simulink model "Decimator"  (R2023b)
settings: Solver=VariableStepAuto  StartTime=0.0  StopTime=18000/(fclk*8)  RelTol=1e-3
PreLoadFcn:
  | startup
values from neighbouring files (symbols this model uses):
  fclk = 64e6    (= 64000000)    [startup.m]
undefined symbols (not defined in the file or in its folder): designMultirateFIR
libraries: hdlBasic x155, dspmlti4 x32, hdlsllib x2, hdlDSPIP x1, dspsrcs4 x1, vmcUtilities x1
settings Model: Creator=andre  LastModifiedBy=andre

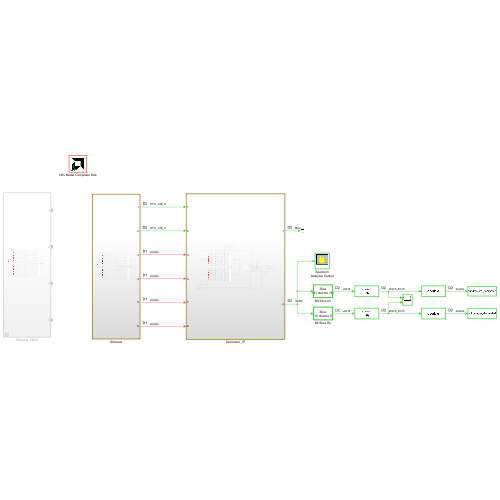
[thumbnail: Simulink's stored preview of the top-level diagram]
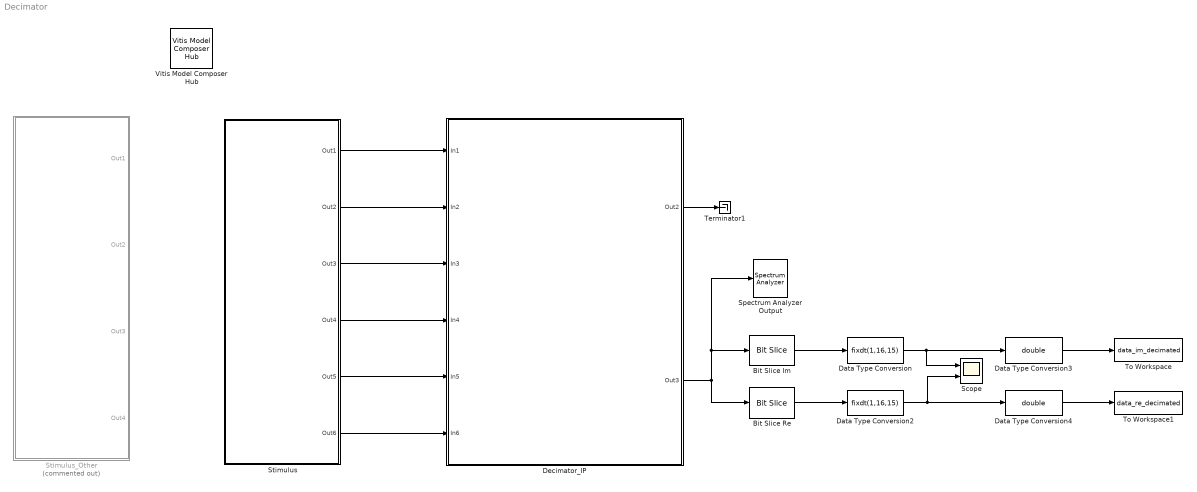
== system Decimator ==
  Bit Slice Im : hdlsllib/Logic and Bit Operations/Bit Slice  lidx=31  ridx=16
  Bit Slice Re : hdlsllib/Logic and Bit Operations/Bit Slice  lidx=15  ridx=0
  Data Type Conversion : DataTypeConversion  OutDataTypeStr=fixdt(1,16,15)  ConvertRealWorld=Stored Integer (SI)  SaturateOnIntegerOverflow=off  RndMeth=Floor
  Data Type Conversion2 : DataTypeConversion  OutDataTypeStr=fixdt(1,16,15)  ConvertRealWorld=Stored Integer (SI)  SaturateOnIntegerOverflow=off  RndMeth=Floor
  Data Type Conversion3 : DataTypeConversion  OutDataTypeStr=double  RndMeth=Floor
  Data Type Conversion4 : DataTypeConversion  OutDataTypeStr=double  RndMeth=Floor
  Decimator_IP : Subsystem
  Scope : Scope  NumInputPorts=2
  Spectrum Analyzer Output : SpectrumAnalyzer  WindowPosition=[2932.000000,-90.000000,799.000000,500.000000,]  ScopeFrameLocation=window  Span=64000000  StartFrequency=-32000000  StopFrequency=32000000  YLimits=[41.6132,126.1267]  SelectedToolstripTab=spectrumAnalyzerToolstrip.measurementsTab
  Stimulus : Subsystem
  Stimulus_Other : Subsystem  Commented=on
  Terminator1 : Terminator
  To Workspace : ToWorkspace  VariableName=data_im_decimated  SaveFormat=Timeseries  SampleTime=-1
  To Workspace1 : ToWorkspace  VariableName=data_re_decimated  SaveFormat=Timeseries  SampleTime=-1
  Vitis Model Composer Hub : vmcUtilities/Vitis Model Composer Hub  Tag=genX  CodeGeneration=off  SubsystemName=Decimator_IP  DUTSubsystemName=Decimator_IP  CompilationType=HDLCompilation  ExportTypeV2=IP Catalog  TargetDirectory=./netlist\ip\Decimator_IP\src  exportDesign=on  analyzeDesign=off  validateDesignOnHw=off  ExportType=HDL  IpVendor=xilinx.com  IpLibrary=hls  IpVersion=1.0  IpHWLanguage=Verilog  AieCompilerOptions={}  AieSimulatorOptions={}  CreateTestbench=off  TestbenchStackSize=10  RunRtlSim=off  RunCSim=off  RunAieSim=off  AieSimTimeout=50000  RunAieSimProfiling=off  LaunchVitisAnalyzer=off  PlotOutput=off  RunX86Sim=off  X86SimTimeout=10  GenHwImage=off  GenLibadfXo=on  GenHwValidationCode=off  PlatformType=Not Specified  HwSystemType=Baremetal  HwValidationTarget=hw  ProjDevice=xczu28dr-ffvg1517-2-e  ProjDevicePart=xczu28dr-ffvg1517-2-e  SamplePeriod=-1  ClockFrequency=200  DataPathParallelism=1  xilinxfamily=zynquplusRFSOC  part=xczu28dr  speed=-2-e  package=ffvg1517  directory=./netlist\ip\Decimator_IP\src  testbench=off  incr_netlist=off  synthesis_tool=Vivado  clock_wrapper=Clock Enables  dbl_ovrd=According to Block Masks  dcm_input_clock_period=10  sysclk_period=(1/fclk)*(1e6)  simulink_period=1/(fclk*8)  eval_field=0  IPInfoJsonString="{\"HDLSubsystem\":{\"SubsystemName\":\"Decimator_IP\",\"IPName\":\"Decimator\",\"IPLibrary\":\"VMC\",\"IPVendor\":\"CoRSoC\",\"IPVersion\":\"1.0\",\"TargetDirectory\":\"./netlist\",\"SubsystemDir\":\"./netlist\\\\ip\\\\Decimator_IP\"},\"SubsystemTag\":\"HDLNode\"}"  LogFileName=''  NThreads=4
  wires:
  Decimator_IP/1(Out2) -> Terminator1/1
  Data Type Conversion3/1 -> To Workspace/1
  Data Type Conversion4/1 -> To Workspace1/1
  Stimulus/1(Out1) -> Decimator_IP/1(In1)
  Stimulus/2(Out2) -> Decimator_IP/2(In2)
  Decimator_IP/2(Out3) -> Bit Slice Im/1, Spectrum Analyzer Output/1, Bit Slice Re/1
  Bit Slice Im/1 -> Data Type Conversion/1
  Bit Slice Re/1 -> Data Type Conversion2/1
  Stimulus/3(Out3) -> Decimator_IP/3(In3)
  Stimulus/4(Out4) -> Decimator_IP/4(In4)
  Data Type Conversion/1 -> Data Type Conversion3/1, Scope/1
  Data Type Conversion2/1 -> Scope/2, Data Type Conversion4/1
  Stimulus/5(Out5) -> Decimator_IP/5(In5)
  Stimulus/6(Out6) -> Decimator_IP/6(In6)

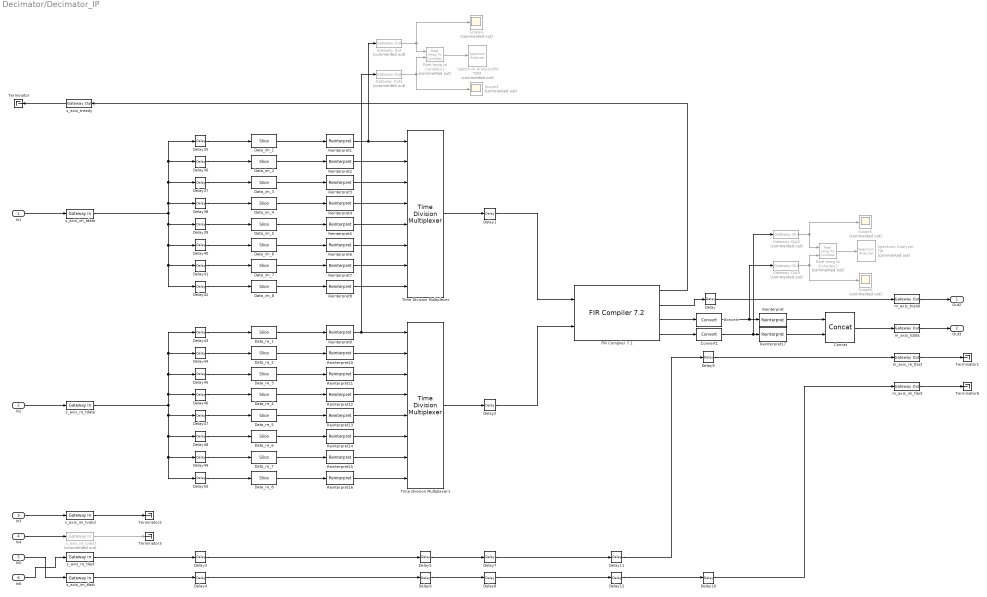
== system Decimator/Decimator_IP ==
  In1 : Inport
  In2 : Inport  Port=2
  In3 : Inport  Port=3
  In4 : Inport  Port=4
  In5 : Inport  Port=5
  In6 : Inport  Port=6
  Concat : hdlBasic/Concat  num_inputs=2  XmcBlockStatus=1  maskContainerNames=group1  block_type=concat  block_config=sysgen:Concat_config
  Convert : hdlBasic/Convert  gui_display_data_type=Fixed-point  arith_type=Signed (2's comp)  n_bits=16  bin_pt=15  float_type=Single  exp_bits=8  fraction_bits=24  quantization=Truncate  overflow=Saturate  en=off  latency=1  pipeline=off  XmcBlockStatus=1  maskContainerNames=group2  block_type=convert  block_config=sysgen:Convert_config  block_width=595  block_height=885
  Convert1 : hdlBasic/Convert  gui_display_data_type=Fixed-point  arith_type=Signed (2's comp)  n_bits=16  bin_pt=15  float_type=Single  exp_bits=8  fraction_bits=24  quantization=Truncate  overflow=Saturate  en=off  latency=1  pipeline=off  XmcBlockStatus=1  maskContainerNames=group2  block_type=convert  block_config=sysgen:Convert_config  block_width=595  block_height=885
  Data_im_1 : hdlBasic/Slice  nbits=16  boolean_output=off  mode=Upper Bit Location + Width  bit1=127  base1=LSB of Input  bit0=16*8-(16*1)  base0=LSB of Input  XmcBlockStatus=1  maskContainerNames=group1  block_type=slice  block_config=sysgen:Slice_config
  Data_im_2 : hdlBasic/Slice  nbits=16  boolean_output=off  mode=Upper Bit Location + Width  bit1=111  base1=LSB of Input  bit0=16*8-(16*1)  base0=LSB of Input  XmcBlockStatus=1  maskContainerNames=group1  block_type=slice  block_config=sysgen:Slice_config
  Data_im_3 : hdlBasic/Slice  nbits=16  boolean_output=off  mode=Upper Bit Location + Width  bit1=95  base1=LSB of Input  bit0=16*8-(16*1)  base0=LSB of Input  XmcBlockStatus=1  maskContainerNames=group1  block_type=slice  block_config=sysgen:Slice_config
  Data_im_4 : hdlBasic/Slice  nbits=16  boolean_output=off  mode=Upper Bit Location + Width  bit1=79  base1=LSB of Input  bit0=16*8-(16*1)  base0=LSB of Input  XmcBlockStatus=1  maskContainerNames=group1  block_type=slice  block_config=sysgen:Slice_config
  Data_im_5 : hdlBasic/Slice  nbits=16  boolean_output=off  mode=Upper Bit Location + Width  bit1=63  base1=LSB of Input  bit0=16*8-(16*1)  base0=LSB of Input  XmcBlockStatus=1  maskContainerNames=group1  block_type=slice  block_config=sysgen:Slice_config
  Data_im_6 : hdlBasic/Slice  nbits=16  boolean_output=off  mode=Upper Bit Location + Width  bit1=47  base1=LSB of Input  bit0=16*8-(16*1)  base0=LSB of Input  XmcBlockStatus=1  maskContainerNames=group1  block_type=slice  block_config=sysgen:Slice_config
  Data_im_7 : hdlBasic/Slice  nbits=16  boolean_output=off  mode=Upper Bit Location + Width  bit1=31  base1=LSB of Input  bit0=16*8-(16*1)  base0=LSB of Input  XmcBlockStatus=1  maskContainerNames=group1  block_type=slice  block_config=sysgen:Slice_config
  Data_im_8 : hdlBasic/Slice  nbits=16  boolean_output=off  mode=Upper Bit Location + Width  bit1=15  base1=LSB of Input  bit0=16*8-(16*1)  base0=LSB of Input  XmcBlockStatus=1  maskContainerNames=group1  block_type=slice  block_config=sysgen:Slice_config
  Data_re_1 : hdlBasic/Slice  nbits=16  boolean_output=off  mode=Upper Bit Location + Width  bit1=127  base1=LSB of Input  bit0=16*8-(16*1)  base0=LSB of Input  XmcBlockStatus=1  maskContainerNames=group1  block_type=slice  block_config=sysgen:Slice_config
  Data_re_2 : hdlBasic/Slice  nbits=16  boolean_output=off  mode=Upper Bit Location + Width  bit1=111  base1=LSB of Input  bit0=16*8-(16*1)  base0=LSB of Input  XmcBlockStatus=1  maskContainerNames=group1  block_type=slice  block_config=sysgen:Slice_config
  Data_re_3 : hdlBasic/Slice  nbits=16  boolean_output=off  mode=Upper Bit Location + Width  bit1=95  base1=LSB of Input  bit0=16*8-(16*1)  base0=LSB of Input  XmcBlockStatus=1  maskContainerNames=group1  block_type=slice  block_config=sysgen:Slice_config
  Data_re_4 : hdlBasic/Slice  nbits=16  boolean_output=off  mode=Upper Bit Location + Width  bit1=79  base1=LSB of Input  bit0=16*8-(16*1)  base0=LSB of Input  XmcBlockStatus=1  maskContainerNames=group1  block_type=slice  block_config=sysgen:Slice_config
  Data_re_5 : hdlBasic/Slice  nbits=16  boolean_output=off  mode=Upper Bit Location + Width  bit1=63  base1=LSB of Input  bit0=16*8-(16*1)  base0=LSB of Input  XmcBlockStatus=1  maskContainerNames=group1  block_type=slice  block_config=sysgen:Slice_config
  Data_re_6 : hdlBasic/Slice  nbits=16  boolean_output=off  mode=Upper Bit Location + Width  bit1=47  base1=LSB of Input  bit0=16*8-(16*1)  base0=LSB of Input  XmcBlockStatus=1  maskContainerNames=group1  block_type=slice  block_config=sysgen:Slice_config
  Data_re_7 : hdlBasic/Slice  nbits=16  boolean_output=off  mode=Upper Bit Location + Width  bit1=31  base1=LSB of Input  bit0=16*8-(16*1)  base0=LSB of Input  XmcBlockStatus=1  maskContainerNames=group1  block_type=slice  block_config=sysgen:Slice_config
  Data_re_8 : hdlBasic/Slice  nbits=16  boolean_output=off  mode=Upper Bit Location + Width  bit1=15  base1=LSB of Input  bit0=16*8-(16*1)  base0=LSB of Input  XmcBlockStatus=1  maskContainerNames=group1  block_type=slice  block_config=sysgen:Slice_config
  Delay{,1..4,7..10,35..50} (25 alike) : hdlBasic/Delay  rst=off  en=off  latency=1  reg_retiming=off  XmcBlockStatus=1  maskContainerNames=group1  block_type=delay  block_config=sysgen:Delay_config
  Delay11 : hdlBasic/Delay  rst=off  en=off  latency=6  reg_retiming=off  XmcBlockStatus=1  maskContainerNames=group1  block_type=delay  block_config=sysgen:Delay_config
  Delay12 : hdlBasic/Delay  rst=off  en=off  latency=6  reg_retiming=off  XmcBlockStatus=1  maskContainerNames=group1  block_type=delay  block_config=sysgen:Delay_config
  Delay5 : hdlBasic/Delay  rst=off  en=off  latency=7  reg_retiming=off  XmcBlockStatus=1  maskContainerNames=group1  block_type=delay  block_config=sysgen:Delay_config
  Delay6 : hdlBasic/Delay  rst=off  en=off  latency=7  reg_retiming=off  XmcBlockStatus=1  maskContainerNames=group1  block_type=delay  block_config=sysgen:Delay_config
  FIR Compiler 7.1 : hdlDSPIP/FIR Compiler 7.2   coefficientvector=coeffs  coefficient_sets=1  coefficient_reload=off  filter_type=Decimation  rate_change_type=Integer  interpolation_rate=1  decimation_rate=8  zero_pack_factor=1  channel_sequence=Basic  number_channels=1  pattern_list='P4-0,P4-1,P4-2,P4-3,P4-4'  number_paths=2  ratespecification=Maximum_Possible  sampleperiod=1  hardwareoversamplingrate=1  coefficient_sign=Signed  quantization=Quantize_Only  coefficient_width=16  bestprecision=on  coefficient_fractional_bits=17  coefficient_structure=Inferred  output_rounding_mode=Full_Precision  output_width=35  filter_architecture=Systolic_Multiply_Accumulate  optimization_goal=Speed  optimization_list='Data_Path_Fanout,Pre-Adder_Pipeline,Coefficient_Fanout,Control_Path_Fanout,Control_Column_Fanout,Control_Broadcast_Fanout,Control_LUT_Pipeline,No_BRAM_Read_First_Mode,Optimal_Column_Lengths,Other'  data_buffer_type=Automatic  coefficient_buffer_type=Automatic  input_buffer_type=Automatic  output_buffer_type=Automatic  preference_for_other_storage=Automatic  multi_column_support=Automatic  columnconfig='15'  inter_column_pipe_length=4  data_has_tlast=Not_Required  m_data_has_tready=off  s_data_has_fifo=off  s_data_has_tuser=Not_Required  m_data_has_tuser=Not_Required  s_config_sync_mode=On_Vector  s_config_method=Single  num_reload_slots=1  has_aclken=off  has_aresetn=off  reset_data_vector=on  trim_axipin_name=on  simulation_type=hybrid_sim  simulation_model=sysgen:xfirv7_2_cmodel  data_path_portlist={ 's_axis_data_tdata', 'm_axis_data_tdata' }  passband_min=0.0  passband_max=0.5  stopband_min=0.5  stopband_max=1.0  filter_selection=1  gui_behaviour='Sysgen_GUI'  data_sign=Signed  data_width=16  data_fractional_bits=0  data_tuser_width=1  wrapper_available=true  ip_wrap_arbitrary_binary_point=true  ip_name=FIR Compiler  ip_version=7.2  dsptool_ready=true  ipcore_usecache=true  ipcore_useipmodelcache=true  port_translation_map={ 'aclken' => 'en', 'aresetn' => 'rst' }  run_core_at_system_period=true  ipcore_xco_need_fpga_part=true  ipcore_fpga_part=[]  XmcBlockStatus=1  maskContainerNames=tabcontainer1  block_type=fir_compiler_v7_2  block_config=sysgen:rodinimport_config  block_width=820  block_height=600
  Gateway Out{,1..3} (4 alike) : hdlBasic/Gateway Out  Commented=on  inherit_from_input=off  hdl_port=off  rows=1  columns=1  UseAsDAC=off  DACChannel='1'  interface=None  automatic_assignment=on  address_offset=hex2dec('00')  intf_name=''  intf_description=''  timing_constraint=None  locs_specified=off  LOCs={}  io_standard={}  XmcBlockStatus=1  maskContainerNames=group4  block_type=gatewayout  block_config=sysgen:gateway_out_config  block_width_w=590  block_height_w=620  block_width=620  block_height=750
  Real-Imag to Complex1 : RealImagToComplex  Commented=on
  Real-Imag to Complex2 : RealImagToComplex  Commented=on
  Reinterpret : hdlBasic/Reinterpret  force_arith_type=on  arith_type=Unsigned  force_bin_pt=on  bin_pt=0  XmcBlockStatus=1  maskContainerNames=group1  block_type=reinterpret  block_config=sysgen:Reinterpret_config
  Reinterpret{1..16} (16 alike) : hdlBasic/Reinterpret  force_arith_type=on  arith_type="Signed  (2's comp)"  force_bin_pt=on  bin_pt=15  XmcBlockStatus=1  maskContainerNames=group1  block_type=reinterpret  block_config=sysgen:Reinterpret_config
  Reinterpret17 : hdlBasic/Reinterpret  force_arith_type=on  arith_type=Unsigned  force_bin_pt=on  bin_pt=0  XmcBlockStatus=1  maskContainerNames=group1  block_type=reinterpret  block_config=sysgen:Reinterpret_config
  Scope{3..6} (4 alike) : Scope  Commented=on
  Spectrum Analyzer FIR : SpectrumAnalyzer  Commented=on  WindowPosition=[481.000000,-215.000000,800.000000,500.000000,]  ScopeFrameLocation=window  Span=64000000  StartFrequency=-32000000  StopFrequency=32000000  YLimits=[-174.72319427,-62.57953967]  SelectedToolstripTab=spectrumAnalyzerToolstrip.measurementsTab
  Spectrum AnalyzerB4 TDM : SpectrumAnalyzer  Commented=on  WindowPosition=[274.000000,72.000000,800.000000,500.000000,]  ScopeFrameLocation=window  Span=512000000  StartFrequency=-256000000  StopFrequency=256000000  YLimits=[-191.4141624,-56.39167641]  SelectedToolstripTab=spectrumAnalyzerToolstrip.measurementsTab
  Terminator{,1..3,6} (5 alike) : Terminator
  Time Division Multiplexer : hdlBasic/Time Division Multiplexer  inputs=8  vin=off  Optimization=Speed  explicit_period=off  period=1  XmcBlockStatus=1  maskContainerNames=group3  block_type=tdm  block_config=sysgen:TDM_config
  Time Division Multiplexer1 : hdlBasic/Time Division Multiplexer  inputs=8  vin=off  Optimization=Speed  explicit_period=off  period=1  XmcBlockStatus=1  maskContainerNames=group3  block_type=tdm  block_config=sysgen:TDM_config
  m_axis_im_tlast : hdlBasic/Gateway Out  inherit_from_input=off  hdl_port=on  rows=1  columns=1  UseAsDAC=off  DACChannel='1'  interface=None  automatic_assignment=on  address_offset=hex2dec('00')  intf_name=''  intf_description=''  timing_constraint=None  locs_specified=off  LOCs={}  io_standard={}  XmcBlockStatus=1  maskContainerNames=group4  block_type=gatewayout  block_config=sysgen:gateway_out_config  block_width_w=590  block_height_w=620  block_width=620  block_height=750
  m_axis_re_tlast : hdlBasic/Gateway Out  inherit_from_input=off  hdl_port=on  rows=1  columns=1  UseAsDAC=off  DACChannel='1'  interface=None  automatic_assignment=on  address_offset=hex2dec('00')  intf_name=''  intf_description=''  timing_constraint=None  locs_specified=off  LOCs={}  io_standard={}  XmcBlockStatus=1  maskContainerNames=group4  block_type=gatewayout  block_config=sysgen:gateway_out_config  block_width_w=590  block_height_w=620  block_width=620  block_height=750
  m_axis_tdata : hdlBasic/Gateway Out  inherit_from_input=on  hdl_port=on  rows=1  columns=1  UseAsDAC=off  DACChannel='1'  interface=None  automatic_assignment=on  address_offset=hex2dec('00')  intf_name=''  intf_description=''  timing_constraint=None  locs_specified=off  LOCs={}  io_standard={}  XmcBlockStatus=1  maskContainerNames=group4  block_type=gatewayout  block_config=sysgen:gateway_out_config  block_width_w=590  block_height_w=620  block_width=620  block_height=750
  m_axis_tvalid : hdlBasic/Gateway Out  inherit_from_input=off  hdl_port=on  rows=1  columns=1  UseAsDAC=off  DACChannel='1'  interface=None  automatic_assignment=on  address_offset=hex2dec('00')  intf_name=''  intf_description=''  timing_constraint=None  locs_specified=off  LOCs={}  io_standard={}  XmcBlockStatus=1  maskContainerNames=group4  block_type=gatewayout  block_config=sysgen:gateway_out_config  block_width_w=590  block_height_w=620  block_width=620  block_height=750
  s_axis_im_tdata : hdlBasic/Gateway In  gui_display_data_type=Fixed-point  arith_type=Unsigned  n_bits=16*8  bin_pt=0  preci_type=Single  exp_width=8  frac_width=24  rows=1  columns=1  quantization=Truncate  overflow=Saturate  period=1/fclk  UseAsADC=off  ADCChannel='1'  interface=None  automatic_assignment=on  address_offset=hex2dec('00')  intf_name=''  intf_description=''  default_value=0  timing_constraint=None  locs_specified=off  LOCs={}  io_standard={}  inherit_from_input=off  hdl_port=on  XmcBlockStatus=1  maskContainerNames=group4  block_type=gatewayin  block_config=sysgen:gateway_in_config  block_width_w=590  block_height_w=620  block_width=640  block_height=850
  s_axis_im_tlast : hdlBasic/Gateway In  gui_display_data_type=Boolean  arith_type=Boolean  n_bits=32  bin_pt=0  preci_type=Single  exp_width=8  frac_width=24  rows=1  columns=1  quantization="Round  (unbiased: +/- Inf)"  overflow=Saturate  period=1/fclk  UseAsADC=off  ADCChannel='1'  interface=None  automatic_assignment=on  address_offset=hex2dec('00')  intf_name=''  intf_description=''  default_value=0  timing_constraint=None  locs_specified=off  LOCs={}  io_standard={}  inherit_from_input=off  hdl_port=on  XmcBlockStatus=1  maskContainerNames=group4  block_type=gatewayin  block_config=sysgen:gateway_in_config  block_width_w=590  block_height_w=620  block_width=640  block_height=850
  s_axis_im_tvalid : hdlBasic/Gateway In  gui_display_data_type=Boolean  arith_type=Boolean  n_bits=32  bin_pt=0  preci_type=Single  exp_width=8  frac_width=24  rows=1  columns=1  quantization="Round  (unbiased: +/- Inf)"  overflow=Saturate  period=1/fclk  UseAsADC=off  ADCChannel='1'  interface=None  automatic_assignment=on  address_offset=hex2dec('00')  intf_name=''  intf_description=''  default_value=0  timing_constraint=None  locs_specified=off  LOCs={}  io_standard={}  inherit_from_input=off  hdl_port=on  XmcBlockStatus=1  maskContainerNames=group4  block_type=gatewayin  block_config=sysgen:gateway_in_config  block_width_w=590  block_height_w=620  block_width=640  block_height=850
  s_axis_re_tdata : hdlBasic/Gateway In  gui_display_data_type=Fixed-point  arith_type=Unsigned  n_bits=16*8  bin_pt=0  preci_type=Single  exp_width=8  frac_width=24  rows=1  columns=1  quantization=Truncate  overflow=Saturate  period=1/fclk  UseAsADC=off  ADCChannel='1'  interface=None  automatic_assignment=on  address_offset=hex2dec('00')  intf_name=''  intf_description=''  default_value=0  timing_constraint=None  locs_specified=off  LOCs={}  io_standard={}  inherit_from_input=off  hdl_port=on  XmcBlockStatus=1  maskContainerNames=group4  block_type=gatewayin  block_config=sysgen:gateway_in_config  block_width_w=590  block_height_w=620  block_width=640  block_height=850
  s_axis_re_tlast : hdlBasic/Gateway In  gui_display_data_type=Boolean  arith_type=Boolean  n_bits=32  bin_pt=0  preci_type=Single  exp_width=8  frac_width=24  rows=1  columns=1  quantization="Round  (unbiased: +/- Inf)"  overflow=Saturate  period=1/fclk  UseAsADC=off  ADCChannel='1'  interface=None  automatic_assignment=on  address_offset=hex2dec('00')  intf_name=''  intf_description=''  default_value=0  timing_constraint=None  locs_specified=off  LOCs={}  io_standard={}  inherit_from_input=off  hdl_port=on  XmcBlockStatus=1  maskContainerNames=group4  block_type=gatewayin  block_config=sysgen:gateway_in_config  block_width_w=590  block_height_w=620  block_width=640  block_height=850
  s_axis_re_tvalid : hdlBasic/Gateway In  Commented=on  gui_display_data_type=Boolean  arith_type=Boolean  n_bits=32  bin_pt=0  preci_type=Single  exp_width=8  frac_width=24  rows=1  columns=1  quantization="Round  (unbiased: +/- Inf)"  overflow=Saturate  period=1/fclk  UseAsADC=off  ADCChannel='1'  interface=None  automatic_assignment=on  address_offset=hex2dec('00')  intf_name=''  intf_description=''  default_value=0  timing_constraint=None  locs_specified=off  LOCs={}  io_standard={}  inherit_from_input=off  hdl_port=on  XmcBlockStatus=1  maskContainerNames=group4  block_type=gatewayin  block_config=sysgen:gateway_in_config  block_width_w=590  block_height_w=620  block_width=640  block_height=850
  s_axis_tready : hdlBasic/Gateway Out  inherit_from_input=off  hdl_port=on  rows=1  columns=1  UseAsDAC=off  DACChannel='1'  interface=None  automatic_assignment=on  address_offset=hex2dec('00')  intf_name=''  intf_description=''  timing_constraint=None  locs_specified=off  LOCs={}  io_standard={}  XmcBlockStatus=1  maskContainerNames=group4  block_type=gatewayout  block_config=sysgen:gateway_out_config  block_width_w=590  block_height_w=620  block_width=620  block_height=750
  Out2 : Outport
  Out3 : Outport  Port=2
  wires:
  In2/1 -> s_axis_re_tdata/1
  In1/1 -> s_axis_im_tdata/1
  FIR Compiler 7.1/2 -> Delay/1
  FIR Compiler 7.1/3 -> Convert/1
  Reinterpret17/1 -> Concat/2
  Convert/1 -> Gateway Out3/1, Reinterpret/1
  FIR Compiler 7.1/1 -> s_axis_tready/1
  Delay/1 -> m_axis_tvalid/1
  Convert1/1 -> Gateway Out2/1, Reinterpret17/1
  Concat/1 -> m_axis_tdata/1
  FIR Compiler 7.1/4 -> Convert1/1
  Reinterpret/1 -> Concat/1
  s_axis_im_tdata/1 -> Delay42/1, Delay41/1, Delay40/1, Delay39/1, Delay38/1, Delay37/1, Delay36/1, Delay35/1
  s_axis_re_tdata/1 -> Delay50/1, Delay49/1, Delay48/1, Delay47/1, Delay46/1, Delay45/1, Delay43/1, Delay44/1
  s_axis_re_tvalid/1 -> Terminator3/1
  s_axis_im_tvalid/1 -> Terminator2/1
  In3/1 -> s_axis_im_tvalid/1
  In4/1 -> s_axis_re_tvalid/1
  s_axis_tready/1 -> Terminator/1
  Time Division Multiplexer/1 -> Delay1/1
  Delay1/1 -> FIR Compiler 7.1/1
  Time Division Multiplexer1/1 -> Delay2/1
  Delay2/1 -> FIR Compiler 7.1/2
  Data_im_1/1 -> Reinterpret1/1
  Data_im_2/1 -> Reinterpret2/1
  Data_im_3/1 -> Reinterpret3/1
  Data_im_4/1 -> Reinterpret4/1
  Data_im_6/1 -> Reinterpret6/1
  Data_im_7/1 -> Reinterpret7/1
  Data_im_8/1 -> Reinterpret8/1
  Data_im_5/1 -> Reinterpret5/1
  Data_re_1/1 -> Reinterpret9/1
  Data_re_3/1 -> Reinterpret11/1
  Data_re_8/1 -> Reinterpret16/1
  Data_re_6/1 -> Reinterpret14/1
  Data_re_7/1 -> Reinterpret15/1
  Data_re_4/1 -> Reinterpret12/1
  Data_re_2/1 -> Reinterpret10/1
  Data_re_5/1 -> Reinterpret13/1
  Reinterpret7/1 -> Time Division Multiplexer/7
  Reinterpret2/1 -> Time Division Multiplexer/2
  Reinterpret8/1 -> Time Division Multiplexer/8
  Reinterpret6/1 -> Time Division Multiplexer/6
  Reinterpret3/1 -> Time Division Multiplexer/3
  Reinterpret4/1 -> Time Division Multiplexer/4
  Reinterpret5/1 -> Time Division Multiplexer/5
  Reinterpret15/1 -> Time Division Multiplexer1/7
  Reinterpret14/1 -> Time Division Multiplexer1/6
  Reinterpret12/1 -> Time Division Multiplexer1/4
  Reinterpret11/1 -> Time Division Multiplexer1/3
  Reinterpret10/1 -> Time Division Multiplexer1/2
  Reinterpret13/1 -> Time Division Multiplexer1/5
  Reinterpret16/1 -> Time Division Multiplexer1/8
  Delay35/1 -> Data_im_1/1
  Delay36/1 -> Data_im_2/1
  Delay37/1 -> Data_im_3/1
  Delay38/1 -> Data_im_4/1
  Delay39/1 -> Data_im_5/1
  Delay40/1 -> Data_im_6/1
  Delay41/1 -> Data_im_7/1
  Delay42/1 -> Data_im_8/1
  Delay43/1 -> Data_re_1/1
  Delay44/1 -> Data_re_2/1
  Delay45/1 -> Data_re_3/1
  Delay46/1 -> Data_re_4/1
  Delay47/1 -> Data_re_5/1
  Delay48/1 -> Data_re_6/1
  Delay49/1 -> Data_re_7/1
  Delay50/1 -> Data_re_8/1
  m_axis_tvalid/1 -> Out2/1
  m_axis_tdata/1 -> Out3/1
  Real-Imag to Complex1/1 -> Spectrum AnalyzerB4 TDM/1
  Reinterpret9/1 -> Time Division Multiplexer1/1, Gateway Out1/1
  Gateway Out/1 -> Scope4/1, Real-Imag to Complex1/1
  Gateway Out1/1 -> Real-Imag to Complex1/2, Scope3/1
  Reinterpret1/1 -> Time Division Multiplexer/1, Gateway Out/1
  Gateway Out2/1 -> Scope5/1, Real-Imag to Complex2/1
  Gateway Out3/1 -> Scope6/1, Real-Imag to Complex2/2
  Real-Imag to Complex2/1 -> Spectrum Analyzer FIR/1
  m_axis_re_tlast/1 -> Terminator1/1
  s_axis_re_tlast/1 -> Delay3/1
  s_axis_im_tlast/1 -> Delay4/1
  m_axis_im_tlast/1 -> Terminator6/1
  In5/1 -> s_axis_im_tlast/1
  In6/1 -> s_axis_re_tlast/1
  Delay3/1 -> Delay5/1
  Delay4/1 -> Delay6/1
  Delay5/1 -> Delay7/1
  Delay6/1 -> Delay8/1
  Delay7/1 -> Delay11/1
  Delay8/1 -> Delay12/1
  Delay9/1 -> m_axis_re_tlast/1
  Delay10/1 -> m_axis_im_tlast/1
  Delay11/1 -> Delay9/1
  Delay12/1 -> Delay10/1

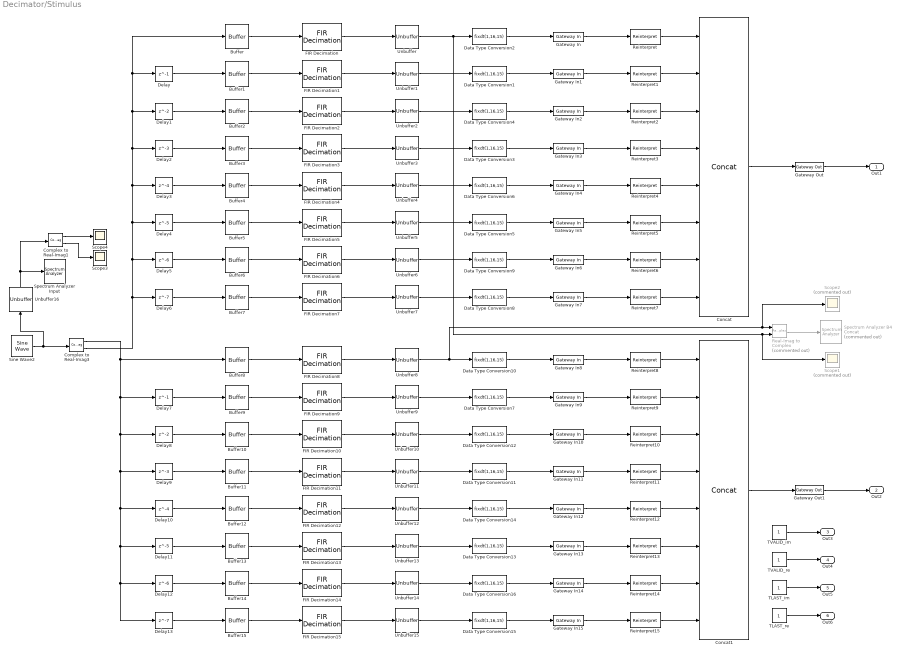
== system Decimator/Stimulus ==
  Buffer{,1..15} (16 alike) : Buffer  OutputFrames=off
  Complex to Real-Imag1 : ComplexToRealImag
  Complex to Real-Imag3 : ComplexToRealImag
  Concat : hdlBasic/Concat  num_inputs=8  XmcBlockStatus=1  maskContainerNames=group1  block_type=concat  block_config=sysgen:Concat_config
  Concat1 : hdlBasic/Concat  num_inputs=8  XmcBlockStatus=1  maskContainerNames=group1  block_type=concat  block_config=sysgen:Concat_config
  Data Type Conversion{1..16} (16 alike) : DataTypeConversion  OutDataTypeStr=fixdt(1,16,15)  RndMeth=Floor
  Delay : Delay  DelayLength=1  InitialCondition=0
  Delay1 : Delay  InitialCondition=0
  Delay10 : Delay  DelayLength=4  InitialCondition=0
  Delay11 : Delay  DelayLength=5  InitialCondition=0
  Delay12 : Delay  DelayLength=6  InitialCondition=0
  Delay13 : Delay  DelayLength=7  InitialCondition=0
  Delay2 : Delay  DelayLength=3  InitialCondition=0
  Delay3 : Delay  DelayLength=4  InitialCondition=0
  Delay4 : Delay  DelayLength=5  InitialCondition=0
  Delay5 : Delay  DelayLength=6  InitialCondition=0
  Delay6 : Delay  DelayLength=7  InitialCondition=0
  Delay7 : Delay  DelayLength=1  InitialCondition=0
  Delay8 : Delay  InitialCondition=0
  Delay9 : Delay  DelayLength=3  InitialCondition=0
  FIR Decimation{,1..15} (16 alike) : dspmlti4/FIR Decimation  FilterSource=Auto  h=designMultirateFIR(1,2)  D=8  filtStruct=Direct form  FilterObject=FDECIM  InputProcessing=Columns as channels (frame based)  framing=Enforce single-rate processing  AllowArbitraryInputLength=off  inputOffset=0  outputBufInitCond=0  roundingMode=Floor  overflowMode=on  firstCoeffDataTypeStr=Inherit: Same word length as input  firstCoeffMin=[]  firstCoeffMax=[]  firstCoeffLastDataTypeStr=Inherit: Same word length as input  outputDataTypeStr=Inherit: Same as accumulator  outputMin=[]  outputMax=[]  outputLastDataTypeStr=Inherit: Same as accumulator
  Gateway In{,1..15} (16 alike) : hdlBasic/Gateway In  gui_display_data_type=Fixed-point  arith_type=Signed (2's comp)  n_bits=16  bin_pt=15  preci_type=Single  exp_width=8  frac_width=24  rows=1  columns=1  quantization=Truncate  overflow=Saturate  period=1/(fclk)  UseAsADC=off  ADCChannel='1'  interface=None  automatic_assignment=on  address_offset=hex2dec('00')  intf_name=''  intf_description=''  default_value=0  timing_constraint=None  locs_specified=off  LOCs={}  io_standard={}  inherit_from_input=off  hdl_port=on  XmcBlockStatus=1  maskContainerNames=group4  block_type=gatewayin  block_config=sysgen:gateway_in_config  block_width_w=590  block_height_w=620  block_width=640  block_height=850
  Gateway Out : hdlBasic/Gateway Out  inherit_from_input=on  hdl_port=off  rows=1  columns=1  UseAsDAC=off  DACChannel='1'  interface=None  automatic_assignment=on  address_offset=hex2dec('00')  intf_name=''  intf_description=''  timing_constraint=None  locs_specified=off  LOCs={}  io_standard={}  XmcBlockStatus=1  maskContainerNames=group4  block_type=gatewayout  block_config=sysgen:gateway_out_config  block_width_w=590  block_height_w=620  block_width=620  block_height=750
  Gateway Out1 : hdlBasic/Gateway Out  inherit_from_input=on  hdl_port=off  rows=1  columns=1  UseAsDAC=off  DACChannel='1'  interface=None  automatic_assignment=on  address_offset=hex2dec('00')  intf_name=''  intf_description=''  timing_constraint=None  locs_specified=off  LOCs={}  io_standard={}  XmcBlockStatus=1  maskContainerNames=group4  block_type=gatewayout  block_config=sysgen:gateway_out_config  block_width_w=590  block_height_w=620  block_width=620  block_height=750
  Real-Imag to Complex : RealImagToComplex  Commented=on
  Reinterpret{,1..15} (16 alike) : hdlBasic/Reinterpret  force_arith_type=on  arith_type=Unsigned  force_bin_pt=on  bin_pt=0  XmcBlockStatus=1  maskContainerNames=group1  block_type=reinterpret  block_config=sysgen:Reinterpret_config
  Scope1 : Scope  Commented=on
  Scope2 : Scope  Commented=on
  Scope3 : Scope
  Scope4 : Scope
  Sine Wave2 : dspsrcs4/Sine Wave  Amplitude=0.9  Frequency=16e6  Phase=0  SampleMode=Discrete  OutComplex=Complex  CompMethod=Trigonometric fcn  TableSize=Speed  SampleTime=1/(fclk*8)  SamplesPerFrame=1  ResetState=Restart at time zero  OutputFrames=off  dataType=double  wordLen=16  udDataType=sfix(16)  fracBitsMode=Best precision  numFracBits=15  OutDataTypeStr=double  LastOutDataTypeStr=double
  Spectrum Analyzer B4 Concat : SpectrumAnalyzer  Commented=on  WindowPosition=[318.000000,62.000000,800.000000,500.000000,]  ScopeFrameLocation=window  Span=512000000  StartFrequency=-256000000  StopFrequency=256000000  YLimits=[-196.33262996,-55.84057964]  SelectedToolstripTab=spectrumAnalyzerToolstrip.measurementsTab
  Spectrum Analyzer Input : SpectrumAnalyzer  WindowPosition=[2124.000000,-89.000000,800.000000,500.000000,]  ScopeFrameLocation=window  Span=512000000  StartFrequency=-256000000  StopFrequency=256000000  YLimits=[-60.80358631,37.98091778]
  TLAST_im : Constant  SampleTime=1/(fclk*8)
  TLAST_re : Constant  SampleTime=1/(fclk*8)
  TVALID_im : Constant  SampleTime=1/(fclk*8)
  TVALID_re : Constant  SampleTime=1/(fclk*8)
  Unbuffer{,1..16} (17 alike) : Unbuffer
  Out1 : Outport
  Out2 : Outport  Port=2
  Out3 : Outport  Port=3
  Out4 : Outport  Port=4
  Out5 : Outport  Port=5
  Out6 : Outport  Port=6
  wires:
  Concat/1 -> Gateway Out/1
  Gateway Out/1 -> Out1/1
  Buffer/1 -> FIR Decimation/1
  Buffer1/1 -> FIR Decimation1/1
  Buffer2/1 -> FIR Decimation2/1
  Buffer3/1 -> FIR Decimation3/1
  Buffer7/1 -> FIR Decimation7/1
  Buffer6/1 -> FIR Decimation6/1
  Buffer5/1 -> FIR Decimation5/1
  Buffer4/1 -> FIR Decimation4/1
  Delay6/1 -> Buffer7/1
  Delay5/1 -> Buffer6/1
  Delay4/1 -> Buffer5/1
  Delay3/1 -> Buffer4/1
  Delay2/1 -> Buffer3/1
  Delay1/1 -> Buffer2/1
  Delay/1 -> Buffer1/1
  FIR Decimation/1 -> Unbuffer/1
  FIR Decimation1/1 -> Unbuffer1/1
  FIR Decimation3/1 -> Unbuffer3/1
  FIR Decimation2/1 -> Unbuffer2/1
  FIR Decimation6/1 -> Unbuffer6/1
  FIR Decimation7/1 -> Unbuffer7/1
  FIR Decimation5/1 -> Unbuffer5/1
  FIR Decimation4/1 -> Unbuffer4/1
  Unbuffer1/1 -> Data Type Conversion1/1
  Unbuffer3/1 -> Data Type Conversion3/1
  Unbuffer2/1 -> Data Type Conversion4/1
  Unbuffer6/1 -> Data Type Conversion9/1
  Unbuffer7/1 -> Data Type Conversion8/1
  Unbuffer5/1 -> Data Type Conversion5/1
  Unbuffer4/1 -> Data Type Conversion6/1
  Data Type Conversion2/1 -> Gateway In/1
  Data Type Conversion1/1 -> Gateway In1/1
  Data Type Conversion3/1 -> Gateway In3/1
  Data Type Conversion4/1 -> Gateway In2/1
  Data Type Conversion9/1 -> Gateway In6/1
  Data Type Conversion8/1 -> Gateway In7/1
  Data Type Conversion5/1 -> Gateway In5/1
  Data Type Conversion6/1 -> Gateway In4/1
  Gateway In1/1 -> Reinterpret1/1
  Gateway In3/1 -> Reinterpret3/1
  Gateway In2/1 -> Reinterpret2/1
  Gateway In6/1 -> Reinterpret6/1
  Gateway In7/1 -> Reinterpret7/1
  Gateway In5/1 -> Reinterpret5/1
  Gateway In4/1 -> Reinterpret4/1
  Reinterpret7/1 -> Concat/8
  Reinterpret1/1 -> Concat/2
  Reinterpret2/1 -> Concat/3
  Reinterpret3/1 -> Concat/4
  Reinterpret4/1 -> Concat/5
  Reinterpret5/1 -> Concat/6
  Reinterpret6/1 -> Concat/7
  Reinterpret14/1 -> Concat1/7
  Reinterpret13/1 -> Concat1/6
  Reinterpret12/1 -> Concat1/5
  Reinterpret11/1 -> Concat1/4
  Reinterpret10/1 -> Concat1/3
  Reinterpret9/1 -> Concat1/2
  Reinterpret15/1 -> Concat1/8
  Gateway In12/1 -> Reinterpret12/1
  Gateway In13/1 -> Reinterpret13/1
  Gateway In15/1 -> Reinterpret15/1
  Gateway In14/1 -> Reinterpret14/1
  Gateway In10/1 -> Reinterpret10/1
  Gateway In11/1 -> Reinterpret11/1
  Gateway In9/1 -> Reinterpret9/1
  Data Type Conversion14/1 -> Gateway In12/1
  Data Type Conversion13/1 -> Gateway In13/1
  Data Type Conversion15/1 -> Gateway In15/1
  Data Type Conversion16/1 -> Gateway In14/1
  Data Type Conversion12/1 -> Gateway In10/1
  Data Type Conversion11/1 -> Gateway In11/1
  Data Type Conversion7/1 -> Gateway In9/1
  Data Type Conversion10/1 -> Gateway In8/1
  Unbuffer12/1 -> Data Type Conversion14/1
  Unbuffer13/1 -> Data Type Conversion13/1
  Unbuffer15/1 -> Data Type Conversion15/1
  Unbuffer14/1 -> Data Type Conversion16/1
  Unbuffer10/1 -> Data Type Conversion12/1
  Unbuffer11/1 -> Data Type Conversion11/1
  Unbuffer9/1 -> Data Type Conversion7/1
  FIR Decimation12/1 -> Unbuffer12/1
  FIR Decimation13/1 -> Unbuffer13/1
  FIR Decimation15/1 -> Unbuffer15/1
  FIR Decimation14/1 -> Unbuffer14/1
  FIR Decimation10/1 -> Unbuffer10/1
  FIR Decimation11/1 -> Unbuffer11/1
  FIR Decimation9/1 -> Unbuffer9/1
  FIR Decimation8/1 -> Unbuffer8/1
  Delay7/1 -> Buffer9/1
  Delay8/1 -> Buffer10/1
  Delay9/1 -> Buffer11/1
  Delay10/1 -> Buffer12/1
  Delay11/1 -> Buffer13/1
  Delay12/1 -> Buffer14/1
  Delay13/1 -> Buffer15/1
  Buffer12/1 -> FIR Decimation12/1
  Buffer13/1 -> FIR Decimation13/1
  Buffer14/1 -> FIR Decimation14/1
  Buffer15/1 -> FIR Decimation15/1
  Buffer11/1 -> FIR Decimation11/1
  Buffer10/1 -> FIR Decimation10/1
  Buffer9/1 -> FIR Decimation9/1
  Buffer8/1 -> FIR Decimation8/1
  Concat1/1 -> Gateway Out1/1
  Reinterpret/1 -> Concat/1
  Gateway In/1 -> Reinterpret/1
  Reinterpret8/1 -> Concat1/1
  Gateway In8/1 -> Reinterpret8/1
  Sine Wave2/1 -> Complex to Real-Imag3/1, Unbuffer16/1
  Gateway Out1/1 -> Out2/1
  TVALID_im/1 -> Out3/1
  TVALID_re/1 -> Out4/1
  Complex to Real-Imag3/2 -> Buffer/1, Delay/1, Delay1/1, Delay2/1, Delay3/1, Delay4/1, Delay5/1, Delay6/1
  Complex to Real-Imag3/1 -> Buffer8/1, Delay10/1, Delay11/1, Delay12/1, Delay13/1, Delay9/1, Delay8/1, Delay7/1
  Real-Imag to Complex/1 -> Spectrum Analyzer B4 Concat/1
  Unbuffer/1 -> Scope1/1, Real-Imag to Complex/2, Data Type Conversion2/1
  Unbuffer8/1 -> Data Type Conversion10/1, Scope2/1, Real-Imag to Complex/1
  Unbuffer16/1 -> Complex to Real-Imag1/1, Spectrum Analyzer Input/1
  Complex to Real-Imag1/1 -> Scope4/1
  Complex to Real-Imag1/2 -> Scope3/1
  TLAST_re/1 -> Out6/1
  TLAST_im/1 -> Out5/1

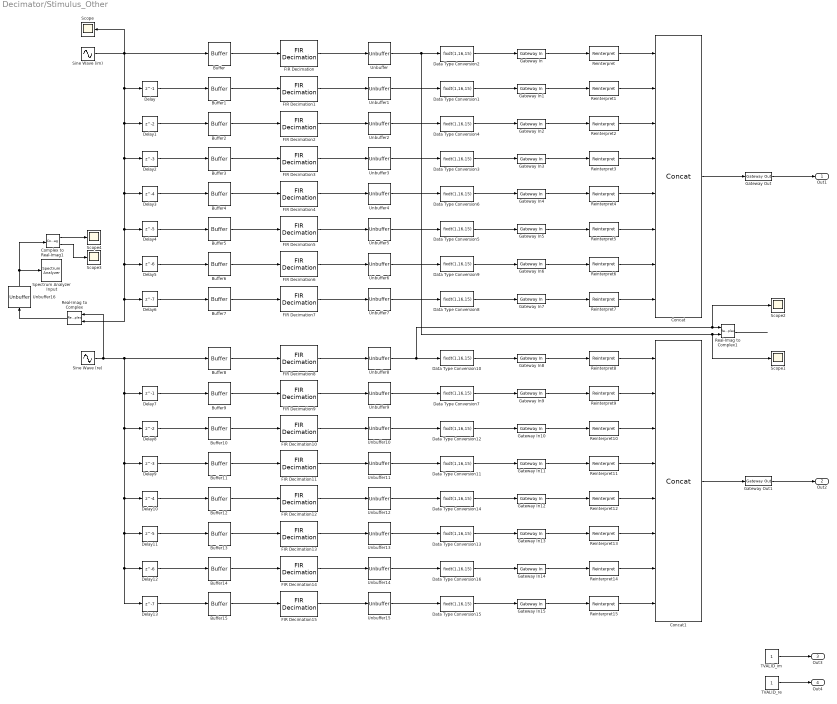
== system Decimator/Stimulus_Other ==
  Buffer{,1..15} (16 alike) : Buffer  OutputFrames=off
  Complex to Real-Imag1 : ComplexToRealImag
  Concat : hdlBasic/Concat  num_inputs=8  XmcBlockStatus=1  maskContainerNames=group1  block_type=concat  block_config=sysgen:Concat_config
  Concat1 : hdlBasic/Concat  num_inputs=8  XmcBlockStatus=1  maskContainerNames=group1  block_type=concat  block_config=sysgen:Concat_config
  Data Type Conversion{1..16} (16 alike) : DataTypeConversion  OutDataTypeStr=fixdt(1,16,15)  RndMeth=Floor
  Delay : Delay  DelayLength=1  InitialCondition=0
  Delay1 : Delay  InitialCondition=0
  Delay10 : Delay  DelayLength=4  InitialCondition=0
  Delay11 : Delay  DelayLength=5  InitialCondition=0
  Delay12 : Delay  DelayLength=6  InitialCondition=0
  Delay13 : Delay  DelayLength=7  InitialCondition=0
  Delay2 : Delay  DelayLength=3  InitialCondition=0
  Delay3 : Delay  DelayLength=4  InitialCondition=0
  Delay4 : Delay  DelayLength=5  InitialCondition=0
  Delay5 : Delay  DelayLength=6  InitialCondition=0
  Delay6 : Delay  DelayLength=7  InitialCondition=0
  Delay7 : Delay  DelayLength=1  InitialCondition=0
  Delay8 : Delay  InitialCondition=0
  Delay9 : Delay  DelayLength=3  InitialCondition=0
  FIR Decimation{,1..15} (16 alike) : dspmlti4/FIR Decimation  FilterSource=Auto  h=designMultirateFIR(1,2)  D=8  filtStruct=Direct form  FilterObject=FDECIM  InputProcessing=Columns as channels (frame based)  framing=Enforce single-rate processing  AllowArbitraryInputLength=off  inputOffset=0  outputBufInitCond=0  roundingMode=Floor  overflowMode=on  firstCoeffDataTypeStr=Inherit: Same word length as input  firstCoeffMin=[]  firstCoeffMax=[]  firstCoeffLastDataTypeStr=Inherit: Same word length as input  outputDataTypeStr=Inherit: Same as accumulator  outputMin=[]  outputMax=[]  outputLastDataTypeStr=Inherit: Same as accumulator
  Gateway In{,1..15} (16 alike) : hdlBasic/Gateway In  gui_display_data_type=Fixed-point  arith_type=Signed (2's comp)  n_bits=16  bin_pt=15  preci_type=Single  exp_width=8  frac_width=24  rows=1  columns=1  quantization=Truncate  overflow=Saturate  period=1/(fclk)  UseAsADC=off  ADCChannel='1'  interface=None  automatic_assignment=on  address_offset=hex2dec('00')  intf_name=''  intf_description=''  default_value=0  timing_constraint=None  locs_specified=off  LOCs={}  io_standard={}  inherit_from_input=off  hdl_port=on  XmcBlockStatus=1  maskContainerNames=group4  block_type=gatewayin  block_config=sysgen:gateway_in_config  block_width_w=590  block_height_w=620  block_width=640  block_height=850
  Gateway Out : hdlBasic/Gateway Out  inherit_from_input=on  hdl_port=off  rows=1  columns=1  UseAsDAC=off  DACChannel='1'  interface=None  automatic_assignment=on  address_offset=hex2dec('00')  intf_name=''  intf_description=''  timing_constraint=None  locs_specified=off  LOCs={}  io_standard={}  XmcBlockStatus=1  maskContainerNames=group4  block_type=gatewayout  block_config=sysgen:gateway_out_config  block_width_w=590  block_height_w=620  block_width=620  block_height=750
  Gateway Out1 : hdlBasic/Gateway Out  inherit_from_input=on  hdl_port=off  rows=1  columns=1  UseAsDAC=off  DACChannel='1'  interface=None  automatic_assignment=on  address_offset=hex2dec('00')  intf_name=''  intf_description=''  timing_constraint=None  locs_specified=off  LOCs={}  io_standard={}  XmcBlockStatus=1  maskContainerNames=group4  block_type=gatewayout  block_config=sysgen:gateway_out_config  block_width_w=590  block_height_w=620  block_width=620  block_height=750
  Real-Imag to Complex : RealImagToComplex
  Real-Imag to Complex1 : RealImagToComplex
  Reinterpret{,1..15} (16 alike) : hdlBasic/Reinterpret  force_arith_type=on  arith_type=Unsigned  force_bin_pt=on  bin_pt=0  XmcBlockStatus=1  maskContainerNames=group1  block_type=reinterpret  block_config=sysgen:Reinterpret_config
  Scope{,1..4} (5 alike) : Scope
  Sine Wave (im) : Sin  Amplitude=.9  Frequency=4e6*pi  SampleTime=1/(fclk*8)
  Sine Wave (re) : Sin  Amplitude=.9  Frequency=4e6*pi  Phase=pi/2  SampleTime=1/(fclk*8)
  Spectrum Analyzer Input : SpectrumAnalyzer  WindowPosition=[182.000000,42.000000,800.000000,500.000000,]  ScopeFrameLocation=window  Span=512000000  StartFrequency=-256000000  StopFrequency=256000000  YLimits=[-60.80358631,37.98091778]  SelectedToolstripTab=spectrumAnalyzerToolstrip.measurementsTab
  TVALID_im : Constant  SampleTime=1/(fclk*8)
  TVALID_re : Constant  SampleTime=1/(fclk*8)
  Unbuffer{,1..16} (17 alike) : Unbuffer
  Out1 : Outport
  Out2 : Outport  Port=2
  Out3 : Outport  Port=3
  Out4 : Outport  Port=4
  wires:
  TVALID_re/1 -> Out4/1
  TVALID_im/1 -> Out3/1
  Gateway Out1/1 -> Out2/1
  Sine Wave (re)/1 -> Buffer8/1, Delay13/1, Delay12/1, Delay11/1, Delay10/1, Delay9/1, Delay8/1, Delay7/1, Real-Imag to Complex/1
  Gateway In8/1 -> Reinterpret8/1
  Reinterpret8/1 -> Concat1/1
  Gateway In/1 -> Reinterpret/1
  Reinterpret/1 -> Concat/1
  Concat1/1 -> Gateway Out1/1
  Buffer8/1 -> FIR Decimation8/1
  Buffer9/1 -> FIR Decimation9/1
  Buffer10/1 -> FIR Decimation10/1
  Buffer11/1 -> FIR Decimation11/1
  Buffer15/1 -> FIR Decimation15/1
  Buffer14/1 -> FIR Decimation14/1
  Buffer13/1 -> FIR Decimation13/1
  Buffer12/1 -> FIR Decimation12/1
  Delay13/1 -> Buffer15/1
  Delay12/1 -> Buffer14/1
  Delay11/1 -> Buffer13/1
  Delay10/1 -> Buffer12/1
  Delay9/1 -> Buffer11/1
  Delay8/1 -> Buffer10/1
  Delay7/1 -> Buffer9/1
  FIR Decimation8/1 -> Unbuffer8/1
  FIR Decimation9/1 -> Unbuffer9/1
  FIR Decimation11/1 -> Unbuffer11/1
  FIR Decimation10/1 -> Unbuffer10/1
  FIR Decimation14/1 -> Unbuffer14/1
  FIR Decimation15/1 -> Unbuffer15/1
  FIR Decimation13/1 -> Unbuffer13/1
  FIR Decimation12/1 -> Unbuffer12/1
  Unbuffer9/1 -> Data Type Conversion7/1
  Unbuffer11/1 -> Data Type Conversion11/1
  Unbuffer10/1 -> Data Type Conversion12/1
  Unbuffer14/1 -> Data Type Conversion16/1
  Unbuffer15/1 -> Data Type Conversion15/1
  Unbuffer13/1 -> Data Type Conversion13/1
  Unbuffer12/1 -> Data Type Conversion14/1
  Data Type Conversion10/1 -> Gateway In8/1
  Data Type Conversion7/1 -> Gateway In9/1
  Data Type Conversion11/1 -> Gateway In11/1
  Data Type Conversion12/1 -> Gateway In10/1
  Data Type Conversion16/1 -> Gateway In14/1
  Data Type Conversion15/1 -> Gateway In15/1
  Data Type Conversion13/1 -> Gateway In13/1
  Data Type Conversion14/1 -> Gateway In12/1
  Gateway In9/1 -> Reinterpret9/1
  Gateway In11/1 -> Reinterpret11/1
  Gateway In10/1 -> Reinterpret10/1
  Gateway In14/1 -> Reinterpret14/1
  Gateway In15/1 -> Reinterpret15/1
  Gateway In13/1 -> Reinterpret13/1
  Gateway In12/1 -> Reinterpret12/1
  Reinterpret15/1 -> Concat1/8
  Reinterpret9/1 -> Concat1/2
  Reinterpret10/1 -> Concat1/3
  Reinterpret11/1 -> Concat1/4
  Reinterpret12/1 -> Concat1/5
  Reinterpret13/1 -> Concat1/6
  Reinterpret14/1 -> Concat1/7
  Reinterpret6/1 -> Concat/7
  Reinterpret5/1 -> Concat/6
  Reinterpret4/1 -> Concat/5
  Reinterpret3/1 -> Concat/4
  Reinterpret2/1 -> Concat/3
  Reinterpret1/1 -> Concat/2
  Reinterpret7/1 -> Concat/8
  Gateway In4/1 -> Reinterpret4/1
  Gateway In5/1 -> Reinterpret5/1
  Gateway In7/1 -> Reinterpret7/1
  Gateway In6/1 -> Reinterpret6/1
  Gateway In2/1 -> Reinterpret2/1
  Gateway In3/1 -> Reinterpret3/1
  Gateway In1/1 -> Reinterpret1/1
  Data Type Conversion6/1 -> Gateway In4/1
  Data Type Conversion5/1 -> Gateway In5/1
  Data Type Conversion8/1 -> Gateway In7/1
  Data Type Conversion9/1 -> Gateway In6/1
  Data Type Conversion4/1 -> Gateway In2/1
  Data Type Conversion3/1 -> Gateway In3/1
  Data Type Conversion1/1 -> Gateway In1/1
  Data Type Conversion2/1 -> Gateway In/1
  Unbuffer4/1 -> Data Type Conversion6/1
  Unbuffer5/1 -> Data Type Conversion5/1
  Unbuffer7/1 -> Data Type Conversion8/1
  Unbuffer6/1 -> Data Type Conversion9/1
  Unbuffer2/1 -> Data Type Conversion4/1
  Unbuffer3/1 -> Data Type Conversion3/1
  Unbuffer1/1 -> Data Type Conversion1/1
  FIR Decimation4/1 -> Unbuffer4/1
  FIR Decimation5/1 -> Unbuffer5/1
  FIR Decimation7/1 -> Unbuffer7/1
  FIR Decimation6/1 -> Unbuffer6/1
  FIR Decimation2/1 -> Unbuffer2/1
  FIR Decimation3/1 -> Unbuffer3/1
  FIR Decimation1/1 -> Unbuffer1/1
  FIR Decimation/1 -> Unbuffer/1
  Delay/1 -> Buffer1/1
  Delay1/1 -> Buffer2/1
  Delay2/1 -> Buffer3/1
  Delay3/1 -> Buffer4/1
  Delay4/1 -> Buffer5/1
  Delay5/1 -> Buffer6/1
  Delay6/1 -> Buffer7/1
  Buffer4/1 -> FIR Decimation4/1
  Buffer5/1 -> FIR Decimation5/1
  Buffer6/1 -> FIR Decimation6/1
  Buffer7/1 -> FIR Decimation7/1
  Buffer3/1 -> FIR Decimation3/1
  Buffer2/1 -> FIR Decimation2/1
  Buffer1/1 -> FIR Decimation1/1
  Buffer/1 -> FIR Decimation/1
  Sine Wave (im)/1 -> Delay/1, Delay1/1, Delay2/1, Delay3/1, Delay4/1, Delay5/1, Real-Imag to Complex/2, Delay6/1, Buffer/1, Scope/1
  Gateway Out/1 -> Out1/1
  Concat/1 -> Gateway Out/1
  Real-Imag to Complex/1 -> Unbuffer16/1
  Real-Imag to Complex1/1 -> ?
  Unbuffer8/1 -> Scope2/1, Real-Imag to Complex1/1, Data Type Conversion10/1
  Unbuffer/1 -> Scope1/1, Real-Imag to Complex1/2, Data Type Conversion2/1
  Complex to Real-Imag1/1 -> Scope4/1
  Complex to Real-Imag1/2 -> Scope3/1
  Unbuffer16/1 -> Complex to Real-Imag1/1, Spectrum Analyzer Input/1
